simulink model "cuadriRotor"  (Simulink 7.5)
settings: Solver=ode3  StartTime=0.0  StopTime=15  FixedStep=0.05  RelTol=1e-3
values from neighbouring files (symbols this model uses):
  b = input('Introduzca b: ')    [practicaCuadriRotor.m]
  x0 = input('Introduzca x0: ')    [practicaCuadriRotor.m]    (also in practicaPVTOL.m)
  xf = input('Introduzca xf: ')    [practicaCuadriRotor.m]    (also in practicaPVTOL.m)
  y0 = input('Introduzca y0: ')    [practicaCuadriRotor.m]    (also in practicaPVTOL.m)
  yf = input('Introduzca yf: ')    [practicaCuadriRotor.m]    (also in practicaPVTOL.m)
  z0 = input('Introduzca z0: ')    [practicaCuadriRotor.m]
  zf = input('Introduzca zf: ')    [practicaCuadriRotor.m]
settings Model: Creator=Celeste Anaid  LastModifiedBy=Mariano
settings OptimizationCC: ExpressionDepthLimit=128
settings DebuggingCC: MultiTaskDSMMsg=warning  MultiTaskCondExecSysMsg=none  FcnCallInpInsideContextMsg=Enable All  StrictBusMsg=None
settings RTWCC: IncludeERTFirstTime=on
settings CodeAppCC: CustomSymbolStrType=$N$R$M_T
settings GRTTargetCC: CombineOutputUpdateFcns=on

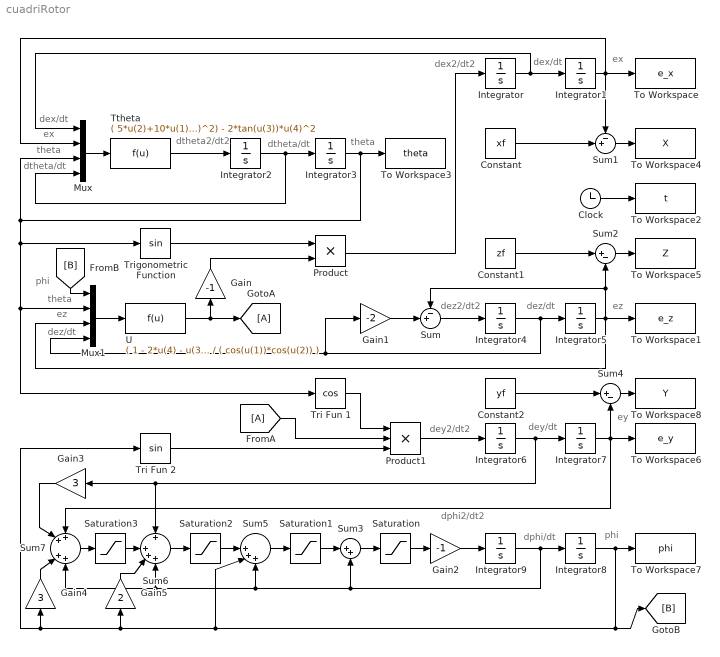
== system cuadriRotor ==
  note: dez/dt
  note: ez
  note: theta
  note: dez/dt
  note: dez2/dt2
  note: theta
  note: dtheta/dt
  note: dtheta2/dt2
  note: theta
  note: dtheta/dt
  note: ex
  note: dex/dt
  note: ex
  note: dex/dt
  note: dex2/dt2
  note: ez
  note: ey
  note: dey/dt
  note: dey2/dt2
  note: phi
  note: phi
  note: dphi/dt
  note: dphi2/dt2
  Clock : Clock
      settings: Decimation=10
  Constant : Constant  Value=xf  OutDataType=fixdt(1, 16)  OutScaling=2^0
  Constant1 : Constant  Value=zf  OutDataType=fixdt(1, 16)  OutScaling=2^0
  Constant2 : Constant  Value=yf  OutDataType=fixdt(1, 16)  OutScaling=2^0
  Gain : Gain  Gain=-1
  Gain1 : Gain  Gain=-2
  Gain2 : Gain  Gain=-1
  Gain3 : Gain  Gain=3  ParameterDataType=fixdt(1, 16)  ParameterScaling=2^0  OutDataType=fixdt(1, 16)  OutScaling=2^0
  Gain4 : Gain  Gain=3  ParameterDataType=fixdt(1, 16)  ParameterScaling=2^0  OutDataType=fixdt(1, 16)  OutScaling=2^0
  Gain5 : Gain  Gain=2  ParameterDataType=fixdt(1, 16)  ParameterScaling=2^0  OutDataType=fixdt(1, 16)  OutScaling=2^0
  Integrator{,2..4,6,8..9} (7 alike) : Integrator
  Integrator1 : Integrator  InitialCondition=xf-x0
  Integrator5 : Integrator  InitialCondition=zf-z0
  Integrator7 : Integrator  InitialCondition=yf-y0
  Mux : Mux
  Mux1 : Mux
  Product : Product
  Product1 : Product  Inputs=3
  Saturation : Saturate  UpperLimit=8*b  LowerLimit=-8*b  OutDataType=fixdt(1, 16)  OutScaling=2^0
  Saturation1 : Saturate  UpperLimit=4*b  LowerLimit=-4*b  OutDataType=fixdt(1, 16)  OutScaling=2^0
  Saturation2 : Saturate  UpperLimit=2*b  LowerLimit=-2*b  OutDataType=fixdt(1, 16)  OutScaling=2^0
  Saturation3 : Saturate  UpperLimit=b  LowerLimit=-b  OutDataType=fixdt(1, 16)  OutScaling=2^0
  Sum : Sum  Inputs=-+|
  Sum1 : Sum  Inputs=-+|  OutDataType=fixdt(1, 16)  OutScaling=2^0
  Sum2 : Sum  Inputs=|+-  OutDataType=fixdt(1, 16)  OutScaling=2^0
  Sum3 : Sum  Inputs=|++  OutDataType=fixdt(1, 16)  OutScaling=2^0
  Sum4 : Sum  Inputs=|+-  OutDataType=fixdt(1, 16)  OutScaling=2^0
  Sum5 : Sum  Inputs=||+++  OutDataType=fixdt(1, 16)  OutScaling=2^0
  Sum6 : Sum  Inputs=+|+++  OutDataType=fixdt(1, 16)  OutScaling=2^0
  Sum7 : Sum  Inputs=++|++  OutDataType=fixdt(1, 16)  OutScaling=2^0
  To Workspace : ToWorkspace  VariableName=e_x  SampleTime=-1  SaveFormat=Array
  To Workspace1 : ToWorkspace  VariableName=e_z  SampleTime=-1  SaveFormat=Array
  To Workspace2 : ToWorkspace  VariableName=t  SampleTime=-1  SaveFormat=Array
  To Workspace3 : ToWorkspace  VariableName=theta  SampleTime=-1  SaveFormat=Array
  To Workspace4 : ToWorkspace  VariableName=X  SampleTime=-1  SaveFormat=Array
  To Workspace5 : ToWorkspace  VariableName=Z  SampleTime=-1  SaveFormat=Array
  To Workspace6 : ToWorkspace  VariableName=e_y  SampleTime=-1  SaveFormat=Array
  To Workspace7 : ToWorkspace  VariableName=phi  SampleTime=-1  SaveFormat=Array
  To Workspace8 : ToWorkspace  VariableName=Y  SampleTime=-1  SaveFormat=Array
  Tri Fun 1 : Trigonometry  Operator=cos
  Tri Fun 2 : Trigonometry
  Trigonometric Function : Trigonometry
  Ttheta : Fcn  Expr=( 5*u(2)+10*u(1)-9*tan(u(3))-4*(1+(tan(u(3))^2))*u(4) )/(1+tan(u(3))^2) - 2*tan(u(3))*u(4)^2
  U : Fcn  Expr=( 1 - 2*u(4) - u(3) ) / ( cos(u(1))*cos(u(2)) )
  wires:
  Integrator/1 -> Integrator1/1, Mux/1
  Integrator1/1 -> To Workspace/1, Sum1/1, Mux/2
  Mux/1 -> Ttheta/1
  Ttheta/1 -> Integrator2/1
  Integrator2/1 -> Integrator3/1, Mux/4
  Integrator3/1 -> To Workspace3/1, Trigonometric Function/1, Tri Fun 1/1, Mux1/2, Mux/3
  Sum/1 -> Integrator4/1
  Mux1/1 -> U/1
  Integrator5/1 -> To Workspace1/1, Sum/1, Sum2/2, Mux1/3
  Clock/1 -> To Workspace2/1
  Integrator4/1 -> Integrator5/1, Gain1/1, Mux1/4
  Gain1/1 -> Sum/2
  Trigonometric Function/1 -> Product/1
  Gain/1 -> Product/2
  Product/1 -> Integrator/1
  Sum1/1 -> To Workspace4/1
  Constant/1 -> Sum1/2
  Sum2/1 -> To Workspace5/1
  Constant1/1 -> Sum2/1
  Integrator6/1 -> Integrator7/1, Gain3/1, Sum6/1
  Integrator7/1 -> Sum4/2, To Workspace6/1, Sum7/1
  Product1/1 -> Integrator6/1
  Tri Fun 1/1 -> Product1/1
  Sum4/1 -> To Workspace8/1
  Constant2/1 -> Sum4/1
  [B] -> Mux1/1
  U/1 -> [A], Gain/1
  Tri Fun 2/1 -> Product1/3
  [A] -> Product1/2
  Integrator8/1 -> To Workspace7/1, [B], Tri Fun 2/1, Gain4/1, Gain5/1, Sum5/2
  Integrator9/1 -> Integrator8/1, Sum3/2, Sum5/3, Sum7/4, Sum6/4
  Gain2/1 -> Integrator9/1
  Saturation/1 -> Gain2/1
  Sum3/1 -> Saturation/1
  Saturation1/1 -> Sum3/1
  Sum5/1 -> Saturation1/1
  Saturation2/1 -> Sum5/1
  Sum6/1 -> Saturation2/1
  Sum7/1 -> Saturation3/1
  Gain3/1 -> Sum7/2
  Gain4/1 -> Sum7/3
  Saturation3/1 -> Sum6/2
  Gain5/1 -> Sum6/3
